simulink model "MD_Flipper"  (R2013a)
settings: Solver=ode45  StartTime=0.0  StopTime=10.0  RelTol=1e-3
libraries: vrlib x2
settings Model: Creator=Armin  LastModifiedBy=Erwin
settings DataIOCC: SignalLoggingSaveFormat=ModelDataLogs
settings OptimizationCC: ExpressionDepthLimit=2147483647
settings DebuggingCC: FcnCallInpInsideContextMsg=UseLocalSettings
settings GRTTargetCC: CombineOutputUpdateFcns=off  GRTInterface=on

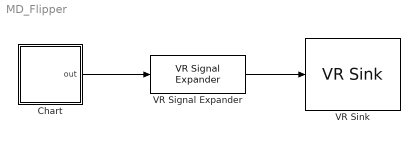
== system MD_Flipper ==
  Chart : Stateflow chart  TreatAsAtomicUnit=on
  VR Signal Expander : vrlib/VR Signal Expander  outwidth=3  outidx=[1 2]
  VR Sink : vrlib/VR Sink  InstantiateOnLoad=on  SampleTime=0.05  ViewEnable=on  RemoteChange=off  RemoteView=on  FieldsWritten=Ball.translation.3.1.1.double  WorldFileName=Table.wrl  AutoView=off  VideoDimensions=[]  AllowVariableSize=off
  wires:
  Chart/1(out) -> VR Signal Expander/1
  VR Signal Expander/1 -> VR Sink/1

== stateflow chart MD_Flipper/Chart ==
  settings: updateMethod=CONTINUOUS
  state Flipper
    during:
    [v_dot[0][0], v_dot[1][0]] = Acc();
    pos_dot = v;
    //Output
    out = pos;
  (default) -> Flipper : {Init();}
  Flipper -> Flipper [order 1] : [WandLinksKontakt()]
      | {WandLinksRefl();}
  Flipper -> Flipper [order 2] : [WandUntenKontakt()]
      | {WandUntenRefl();}
  Flipper -> Flipper [order 3] : [WandRechtsKontakt()]
      | {WandRechtsRefl();}
  Flipper -> Flipper [order 4] : [HndKontakt()]
      | {HndRefl();}
  data: ax function_output double; ay function_output double; k function_output boolean; k function_output boolean; k function_output boolean; k function_output boolean; out output double size=2,1; pos local double size=2,1; v local double size=2,1; p2 local double size=2,1; p1 local double size=2,1; p3 local double size=2,1; p4 local double size=2,1; n_unten local double size=2,1; R constant double =0.25; t_unten local double size=2,1; n_links local double size=2,1; t_links local double size=2,1; n_rechts local double size=2,1; t_rechts local double size=2,1; hnd local double size=2,1; RHnd constant double =0.8
  data pos settings: updateMethod=SF_CONTINUOUS_TIME_DATA
  data v settings: updateMethod=SF_CONTINUOUS_TIME_DATA
  function [ax, ay] =  Acc:
    | function [ax, ay] =  Acc
    | ax = 0; ay = -1;
  function Init:
    | function Init
    |     %Hindernis
    | 	hnd=[6;2.5];
    |     
    |     %Waende
    | 	p1=[0;5];
    | 	p2=[5;0];
    | 	p3=[9;0];
    | 	p4=[10;7];
    |     
    |     %Startposition und Geschwindigkeit
    | 	pos=[4;5]; 
    | 	v=[0;0];
    | 	
    | 	%Einheitsvektoren Normalen- u. Tangentialenrichtung
    | 	t_links=(p2-p1)/norm(p2-p1);
    | 	n_links=[-t_links(2,1); t_links(1,1)];
    | 	t_unten=(p3-p2)/norm(p3-p2);
    | 	n_unten=[-t_unten(2,1); t_unten(1,1)];
    | 	t_rechts=(p4-p3)/norm(p4-p3);
    | 	n_rechts=[-t_rechts(2,1); t_rechts(1,1)];
  function k = WandUntenKontakt:
    | %Testen ob die Kugel die Wand berührt
    | function k = WandUntenKontakt
    | 	k = ((pos-p2)' * n_unten) <= R;
  function WandUntenRefl:
    | %Reflexion nach Kontakt
    | function WandUntenRefl
    | 	vt=v' * t_unten;
    | 	vn=v' * n_unten;
    | 	
    | 	%Neue Geschwindigkeit
    | 	v=vt*t_unten-vn*n_unten;
  function k = WandLinksKontakt:
    | %Testen ob die Kugel die Wand berührt
    | function k = WandLinksKontakt
    |     k = ((pos-p1)' * n_links) <= R;
  function WandLinksRefl:
    | %Reflexion nach Kontakt
    | function WandLinksRefl
    | 	vt=v' * t_links;
    | 	vn=v' * n_links;
    | 	
    | 	%Neue Geschwindigkeit
    | 	v=vt*t_links-vn*n_links;
  function k = WandRechtsKontakt:
    | %Testen ob die Kugel die Wand berührt
    | function k = WandRechtsKontakt
    |     k = ((pos-p3)' * n_rechts) <= R;
  function WandRechtsRefl:
    | %Reflexion nach Kontakt
    | function WandRechtsRefl
    | 	vt=v' * t_rechts;
    | 	vn=v' * n_rechts;
    | 	
    | 	%Neue Geschwindigkeit
    | 	v=vt*t_rechts-vn*n_rechts;
  function k = HndKontakt:
    | %Testen ob die Kugel das Hindernis berührt
    | function k = HndKontakt
    | 	k = (norm(pos-hnd)) <= R + RHnd;
  function HndRefl:
    | %Reflexion nach Kontakt
    | function HndRefl
    | 	n=(pos-hnd)/norm(pos-hnd);
    | 	t=[n(2,1); -n(1,1)];
    | 	
    | 	%Neue Geschwindigkeit
    | 	vt=v'*t;
    | 	vn=v'*n;
    | 	v=vt*t-vn*n;
